simulink model "inputshaping_lab"  (R2023b)
settings: Solver=ode5  StartTime=0.0  StopTime=20  RelTol=1e-3
values from neighbouring files (symbols this model uses):
  SampleTime = 0.01    [responses0704.m]
undefined symbols (not defined in the file or in its folder): National_Instruments, PCI
libraries: sldrtlib x24, SignalEditorBlockLib x3
settings Model: Creator=labadmin  LastModifiedBy=labadmin
settings HardwareCC: ProdBitPerLong=64  ProdHWDeviceType=Intel->x86-64 (Linux 64)
settings RTWCC: Description=Simulink Desktop Real-Time  SystemTargetFile=sldrt.tlc  TemplateMakefile=sldrt.tmf  RTWCompilerOptimization=on
settings CodeAppCC: MaxIdLength=95
settings SimulinkDesktopRealTimeCC: TargetLibSuffix=_sldrt.a  TargetPreCompLibLocation=C:\Program Files\MATLAB\R2023b\toolbox\sldrt\lib\win64

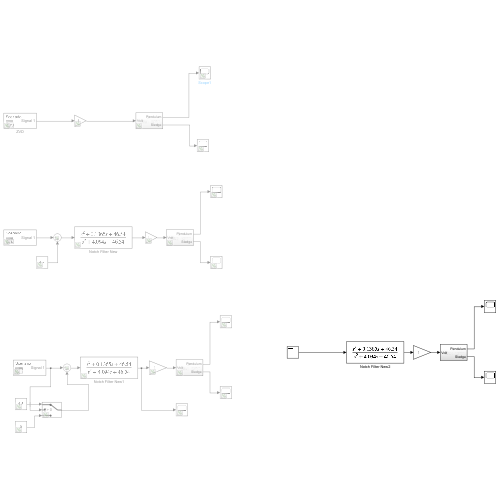
[thumbnail: Simulink's stored preview of the top-level diagram]
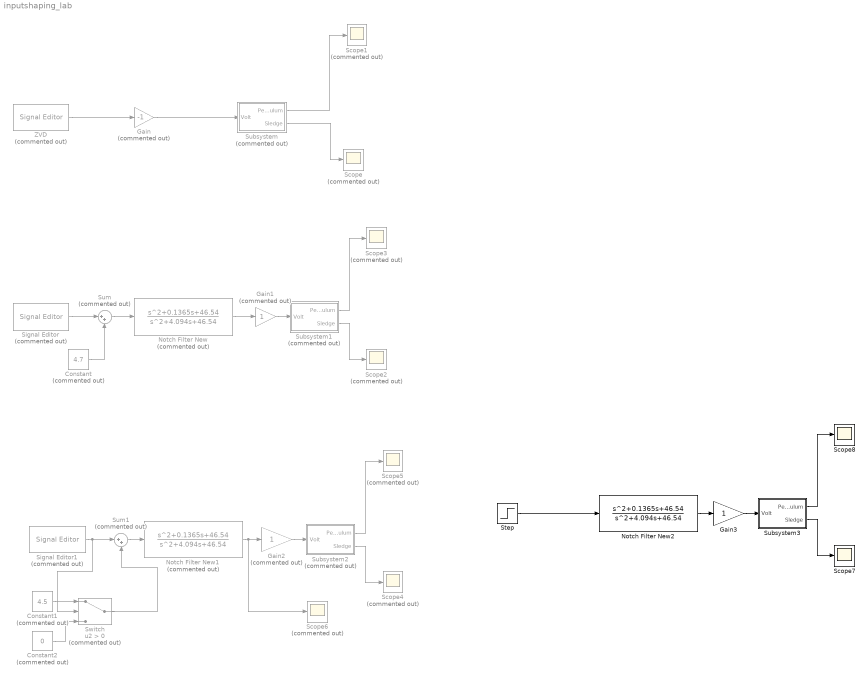
== system inputshaping_lab ==
  Constant : Constant  Commented=on  Value=4.7
  Constant1 : Constant  Commented=on  Value=4.5
  Constant2 : Constant  Commented=on  Value=0
  Gain : Gain  Commented=on  Gain=-1
  Gain1 : Gain  Commented=on
  Gain2 : Gain  Commented=on
  Gain3 : Gain
  Notch Filter New : TransferFcn  Commented=on  Numerator=[1 0.1365 46.54]  Denominator=[1 4.094 46.54]
  Notch Filter New1 : TransferFcn  Commented=on  Numerator=[1 0.1365 46.54]  Denominator=[1 4.094 46.54]
  Notch Filter New2 : TransferFcn  Numerator=[1 0.1365 46.54]  Denominator=[1 4.094 46.54]
  Scope{,1..6} (7 alike) : Scope  Commented=on
  Scope7 : Scope
  Scope8 : Scope
  Signal Editor : SignalEditorBlockLib/Signal Editor  Commented=on  FileName=ZV.mat  ActiveScenario=Scenario  ActiveSignal=Signal 1  IsBus=off  OutputBusObjectStr=Bus: BusObject  SampleTime=0  ZeroCross=off  OutputAfterFinalValue=Setting to zero  Unit=inherit  PreserveSignalName=on  ApplySigPropsToAllScenarios=on  ApplySigPropsToAllSignals=off
  Signal Editor1 : SignalEditorBlockLib/Signal Editor  Commented=on  FileName=ZV.mat  ActiveScenario=Scenario  ActiveSignal=Signal 1  IsBus=off  OutputBusObjectStr=Bus: BusObject  SampleTime=0  ZeroCross=off  OutputAfterFinalValue=Setting to zero  Unit=inherit  PreserveSignalName=on  ApplySigPropsToAllScenarios=on  ApplySigPropsToAllSignals=off
  Step : Step  Time=1.2  Before=9  After=0  SampleTime=0
  Subsystem : Subsystem  Commented=on
  Subsystem1 : Subsystem  Commented=on
  Subsystem2 : Subsystem  Commented=on
  Subsystem3 : Subsystem
  Sum : Sum  Commented=on  Inputs=|++
  Sum1 : Sum  Commented=on  Inputs=|++
  Switch : Switch  Commented=on  Criteria=u2 > Threshold  SaturateOnIntegerOverflow=off  InputSameDT=off
  ZVD : SignalEditorBlockLib/Signal Editor  Commented=on  FileName=signal_input2.mat  ActiveScenario=Scenario  ActiveSignal=Signal 1  IsBus=off  OutputBusObjectStr=Bus: BusObject  SampleTime=0  ZeroCross=off  OutputAfterFinalValue=Setting to zero  Unit=inherit  PreserveSignalName=on  ApplySigPropsToAllScenarios=on  ApplySigPropsToAllSignals=off
  wires:
  ZVD/1 -> Gain/1
  Signal Editor/1 -> Sum/1
  Subsystem/1(Pendulum) -> Scope1/1
  Subsystem/2(Sledge) -> Scope/1
  Gain/1 -> Subsystem/1(Volt)
  Notch Filter New/1 -> Gain1/1
  Subsystem1/1(Pendulum) -> Scope3/1
  Subsystem1/2(Sledge) -> Scope2/1
  Sum/1 -> Notch Filter New/1
  Constant/1 -> Sum/2
  Gain1/1 -> Subsystem1/1(Volt)
  Switch/1 -> Sum1/2
  Subsystem2/2(Sledge) -> Scope4/1
  Signal Editor1/1 -> Switch/2, Sum1/1
  Sum1/1 -> Notch Filter New1/1
  Subsystem2/1(Pendulum) -> Scope5/1
  Gain2/1 -> Subsystem2/1(Volt)
  Constant1/1 -> Switch/1
  Constant2/1 -> Switch/3
  Gain3/1 -> Subsystem3/1(Volt)
  Subsystem3/2(Sledge) -> Scope7/1
  Subsystem3/1(Pendulum) -> Scope8/1
  Step/1 -> Notch Filter New2/1
  Notch Filter New1/1 -> Scope6/1, Gain2/1
  Notch Filter New2/1 -> Gain3/1

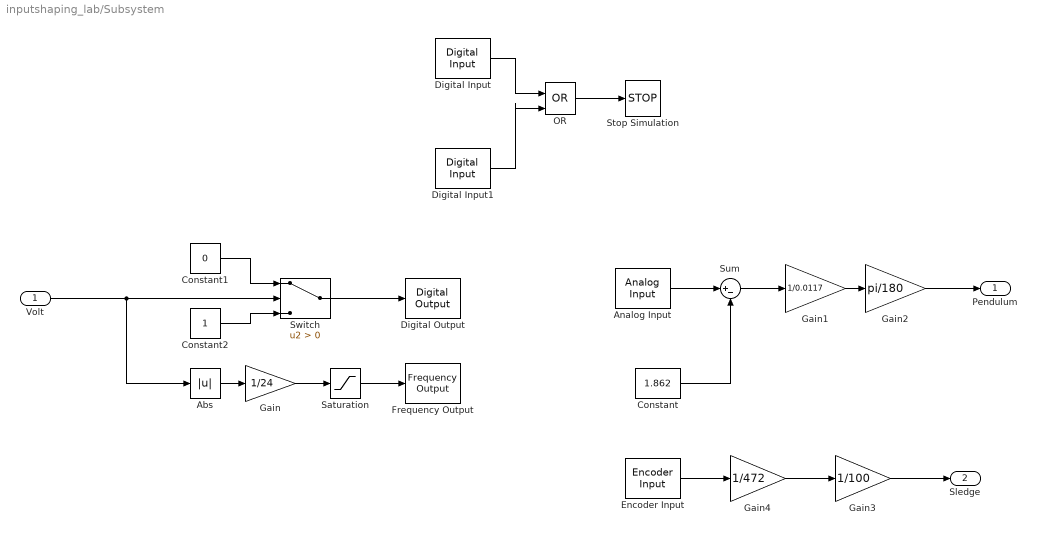
== system inputshaping_lab/Subsystem ==
  Volt : Inport
  Abs : Abs  SaturateOnIntegerOverflow=off
  Analog Input : sldrtlib/Analog Input  SampleTime=-1  MaxMissedTicks=1000000000  ShowMissedTicks=off  YieldWhenWaiting=off  DrvName=National_Instruments/PCI-6229  DrvAddress=4294967295  DrvOptions=[0 1 8192 2 3]  Channels=1  RangeMode=1  VoltRange=1  DataType=1
      settings: AttributesFormatString=National Instruments\nPCI-6229 [auto]
  Constant : Constant  Value=1.862
  Constant1 : Constant  Value=0
  Constant2 : Constant
  Digital Input : sldrtlib/Digital Input  SampleTime=0.1  MaxMissedTicks=10  ShowMissedTicks=off  YieldWhenWaiting=off  DrvName=National_Instruments/PCI-6229  DrvAddress=0  DrvOptions=[1 1 8192 2 3]  Channels=3  BitMode=1  DataType=1
      settings: AttributesFormatString=National Instruments\nPCI-6229 [0]
  Digital Input1 : sldrtlib/Digital Input  SampleTime=0.1  MaxMissedTicks=10  ShowMissedTicks=off  YieldWhenWaiting=off  DrvName=National_Instruments/PCI-6229  DrvAddress=0  DrvOptions=[1 1 8192 2 3]  Channels=2  BitMode=1  DataType=1
      settings: AttributesFormatString=National Instruments\nPCI-6229 [0]
  Digital Output : sldrtlib/Digital Output  SampleTime=-1  MaxMissedTicks=100000000  ShowMissedTicks=off  YieldWhenWaiting=off  DrvName=National_Instruments/PCI-6229  DrvAddress=4294967295  DrvOptions=[0 1 8192 2 3]  Channels=1  BitMode=1  InitialValue=[]  FinalValue=[]
      settings: AttributesFormatString=National Instruments\nPCI-6229 [auto]
  Encoder Input : sldrtlib/Encoder Input  SampleTime=-1  MaxMissedTicks=10000000  ShowMissedTicks=off  YieldWhenWaiting=off  DrvName=National_Instruments/PCI-6229  DrvAddress=4294967295  DrvOptions=[0 1 8192 2 3]  Channels=1  QuadMode=3  IndexPulse=2  InputFilter=Inf  DataType=1
      settings: AttributesFormatString=National Instruments\nPCI-6229 [auto]
  Frequency Output : sldrtlib/Frequency Output  SampleTime=-1  MaxMissedTicks=1000000000  ShowMissedTicks=off  YieldWhenWaiting=off  DrvName=National_Instruments/PCI-6229  DrvAddress=4294967295  DrvOptions=[0 1 8192 2 3]  Channels=2  FrequencySource=1  Frequency=10000  FrequencyFinalValue=[]  DutySource=2  Duty=0  DutyFinalValue=0
      settings: AttributesFormatString=National Instruments\nPCI-6229 [auto]
  Gain : Gain  Gain=1/24
  Gain1 : Gain  Gain=1/0.0117
  Gain2 : Gain  Gain=pi/180
  Gain3 : Gain  Gain=1/100
  Gain4 : Gain  Gain=1/472
  OR : Logic  Operator=OR  IconShape=distinctive  AllPortsSameDT=off  OutDataTypeStr=boolean
  Saturation : Saturate  LowerLimit=0
  Stop Simulation : Stop
  Sum : Sum  Inputs=|+-
  Switch : Switch  Criteria=u2 > Threshold  SaturateOnIntegerOverflow=off  InputSameDT=off
  Pendulum : Outport  VectorParamsAs1DForOutWhenUnconnected=off
  Sledge : Outport  Port=2  VectorParamsAs1DForOutWhenUnconnected=off
  wires:
  Abs/1 -> Gain/1
  Analog Input/1 -> Sum/1
  Gain/1 -> Saturation/1
  Volt/1 -> Abs/1, Switch/2
  Constant2/1 -> Switch/3
  Constant1/1 -> Switch/1
  Switch/1 -> Digital Output/1
  Encoder Input/1 -> Gain4/1
  Saturation/1 -> Frequency Output/1
  Sum/1 -> Gain1/1
  Gain3/1 -> Sledge/1
  Gain4/1 -> Gain3/1
  Constant/1 -> Sum/2
  Gain1/1 -> Gain2/1
  Gain2/1 -> Pendulum/1
  Digital Input1/1 -> OR/2
  Digital Input/1 -> OR/1
  OR/1 -> Stop Simulation/1

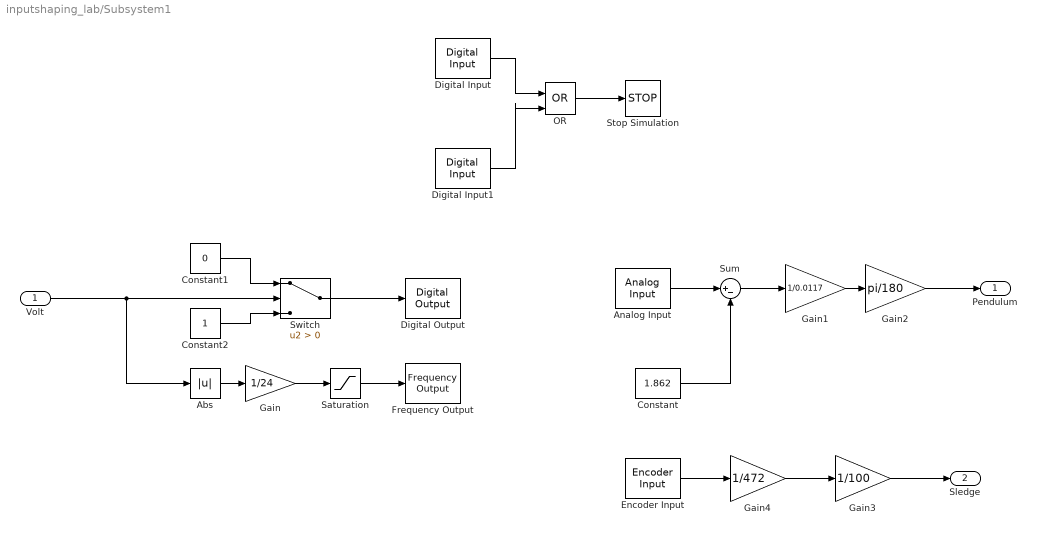
== system inputshaping_lab/Subsystem1 ==
  Volt : Inport
  Abs : Abs  SaturateOnIntegerOverflow=off
  Analog Input : sldrtlib/Analog Input  SampleTime=SampleTime  MaxMissedTicks=MaxMissedTicks  ShowMissedTicks=off  YieldWhenWaiting=off  DrvName=National_Instruments/PCI-6229  DrvAddress=4294967295  DrvOptions=[0 1 8192 2 3]  Channels=1  RangeMode=1  VoltRange=1  DataType=1
      settings: AttributesFormatString=National Instruments\nPCI-6229 [auto]
  Constant : Constant  Value=1.862
  Constant1 : Constant  Value=0
  Constant2 : Constant
  Digital Input : sldrtlib/Digital Input  SampleTime=0.1  MaxMissedTicks=10  ShowMissedTicks=off  YieldWhenWaiting=off  DrvName=National_Instruments/PCI-6229  DrvAddress=0  DrvOptions=[1 1 8192 2 3]  Channels=3  BitMode=1  DataType=1
      settings: AttributesFormatString=National Instruments\nPCI-6229 [0]
  Digital Input1 : sldrtlib/Digital Input  SampleTime=0.1  MaxMissedTicks=10  ShowMissedTicks=off  YieldWhenWaiting=off  DrvName=National_Instruments/PCI-6229  DrvAddress=0  DrvOptions=[1 1 8192 2 3]  Channels=2  BitMode=1  DataType=1
      settings: AttributesFormatString=National Instruments\nPCI-6229 [0]
  Digital Output : sldrtlib/Digital Output  SampleTime=SampleTime  MaxMissedTicks=MaxMissedTicks  ShowMissedTicks=off  YieldWhenWaiting=off  DrvName=National_Instruments/PCI-6229  DrvAddress=4294967295  DrvOptions=[0 1 8192 2 3]  Channels=1  BitMode=1  InitialValue=[]  FinalValue=[]
      settings: AttributesFormatString=National Instruments\nPCI-6229 [auto]
  Encoder Input : sldrtlib/Encoder Input  SampleTime=SampleTime  MaxMissedTicks=MaxMissedTicks  ShowMissedTicks=off  YieldWhenWaiting=off  DrvName=National_Instruments/PCI-6229  DrvAddress=4294967295  DrvOptions=[0 1 8192 2 3]  Channels=1  QuadMode=3  IndexPulse=2  InputFilter=Inf  DataType=1
      settings: AttributesFormatString=National Instruments\nPCI-6229 [auto]
  Frequency Output : sldrtlib/Frequency Output  SampleTime=SampleTime  MaxMissedTicks=MaxMissedTicks  ShowMissedTicks=off  YieldWhenWaiting=off  DrvName=National_Instruments/PCI-6229  DrvAddress=4294967295  DrvOptions=[0 1 8192 2 3]  Channels=2  FrequencySource=1  Frequency=10000  FrequencyFinalValue=[]  DutySource=2  Duty=0  DutyFinalValue=0
      settings: AttributesFormatString=National Instruments\nPCI-6229 [auto]
  Gain : Gain  Gain=1/24
  Gain1 : Gain  Gain=1/0.0117
  Gain2 : Gain  Gain=pi/180
  Gain3 : Gain  Gain=1/100
  Gain4 : Gain  Gain=1/472
  OR : Logic  Operator=OR  IconShape=distinctive  AllPortsSameDT=off  OutDataTypeStr=boolean
  Saturation : Saturate  LowerLimit=0
  Stop Simulation : Stop
  Sum : Sum  Inputs=|+-
  Switch : Switch  Criteria=u2 > Threshold  SaturateOnIntegerOverflow=off  InputSameDT=off
  Pendulum : Outport  VectorParamsAs1DForOutWhenUnconnected=off
  Sledge : Outport  Port=2  VectorParamsAs1DForOutWhenUnconnected=off
  wires:
  Abs/1 -> Gain/1
  Analog Input/1 -> Sum/1
  Gain/1 -> Saturation/1
  Volt/1 -> Abs/1, Switch/2
  Constant2/1 -> Switch/3
  Constant1/1 -> Switch/1
  Switch/1 -> Digital Output/1
  Encoder Input/1 -> Gain4/1
  Saturation/1 -> Frequency Output/1
  Sum/1 -> Gain1/1
  Gain3/1 -> Sledge/1
  Gain4/1 -> Gain3/1
  Constant/1 -> Sum/2
  Gain1/1 -> Gain2/1
  Gain2/1 -> Pendulum/1
  Digital Input1/1 -> OR/2
  Digital Input/1 -> OR/1
  OR/1 -> Stop Simulation/1

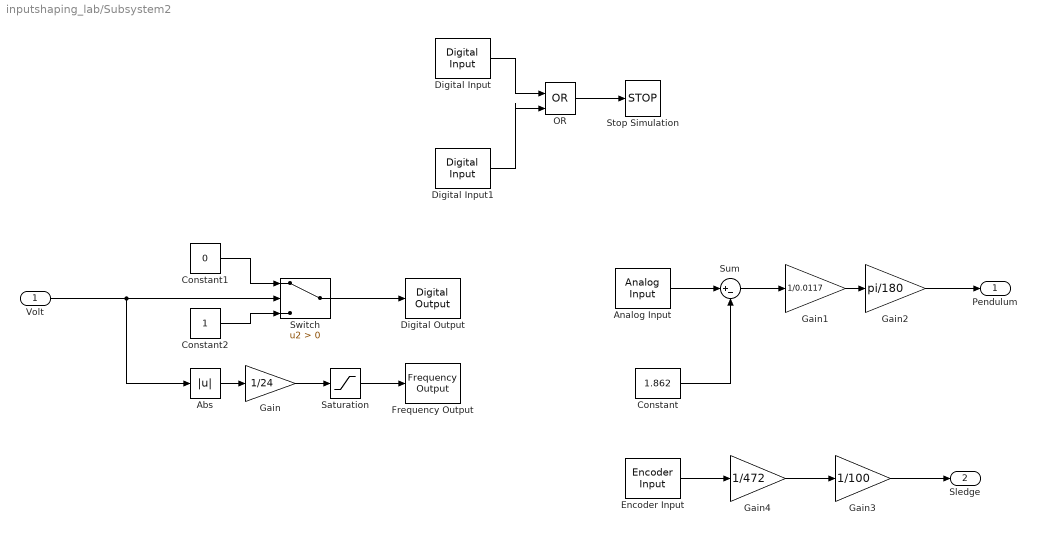
== system inputshaping_lab/Subsystem2 ==
  Volt : Inport
  Abs : Abs  SaturateOnIntegerOverflow=off
  Analog Input : sldrtlib/Analog Input  SampleTime=SampleTime  MaxMissedTicks=MaxMissedTicks  ShowMissedTicks=off  YieldWhenWaiting=off  DrvName=National_Instruments/PCI-6229  DrvAddress=4294967295  DrvOptions=[0 1 8192 2 3]  Channels=1  RangeMode=1  VoltRange=1  DataType=1
      settings: AttributesFormatString=National Instruments\nPCI-6229 [auto]
  Constant : Constant  Value=1.862
  Constant1 : Constant  Value=0
  Constant2 : Constant
  Digital Input : sldrtlib/Digital Input  SampleTime=0.1  MaxMissedTicks=10  ShowMissedTicks=off  YieldWhenWaiting=off  DrvName=National_Instruments/PCI-6229  DrvAddress=0  DrvOptions=[1 1 8192 2 3]  Channels=3  BitMode=1  DataType=1
      settings: AttributesFormatString=National Instruments\nPCI-6229 [0]
  Digital Input1 : sldrtlib/Digital Input  SampleTime=0.1  MaxMissedTicks=10  ShowMissedTicks=off  YieldWhenWaiting=off  DrvName=National_Instruments/PCI-6229  DrvAddress=0  DrvOptions=[1 1 8192 2 3]  Channels=2  BitMode=1  DataType=1
      settings: AttributesFormatString=National Instruments\nPCI-6229 [0]
  Digital Output : sldrtlib/Digital Output  SampleTime=SampleTime  MaxMissedTicks=MaxMissedTicks  ShowMissedTicks=off  YieldWhenWaiting=off  DrvName=National_Instruments/PCI-6229  DrvAddress=4294967295  DrvOptions=[0 1 8192 2 3]  Channels=1  BitMode=1  InitialValue=[]  FinalValue=[]
      settings: AttributesFormatString=National Instruments\nPCI-6229 [auto]
  Encoder Input : sldrtlib/Encoder Input  SampleTime=SampleTime  MaxMissedTicks=MaxMissedTicks  ShowMissedTicks=off  YieldWhenWaiting=off  DrvName=National_Instruments/PCI-6229  DrvAddress=4294967295  DrvOptions=[0 1 8192 2 3]  Channels=1  QuadMode=3  IndexPulse=2  InputFilter=Inf  DataType=1
      settings: AttributesFormatString=National Instruments\nPCI-6229 [auto]
  Frequency Output : sldrtlib/Frequency Output  SampleTime=SampleTime  MaxMissedTicks=MaxMissedTicks  ShowMissedTicks=off  YieldWhenWaiting=off  DrvName=National_Instruments/PCI-6229  DrvAddress=4294967295  DrvOptions=[0 1 8192 2 3]  Channels=2  FrequencySource=1  Frequency=10000  FrequencyFinalValue=[]  DutySource=2  Duty=0  DutyFinalValue=0
      settings: AttributesFormatString=National Instruments\nPCI-6229 [auto]
  Gain : Gain  Gain=1/24
  Gain1 : Gain  Gain=1/0.0117
  Gain2 : Gain  Gain=pi/180
  Gain3 : Gain  Gain=1/100
  Gain4 : Gain  Gain=1/472
  OR : Logic  Operator=OR  IconShape=distinctive  AllPortsSameDT=off  OutDataTypeStr=boolean
  Saturation : Saturate  LowerLimit=0
  Stop Simulation : Stop
  Sum : Sum  Inputs=|+-
  Switch : Switch  Criteria=u2 > Threshold  SaturateOnIntegerOverflow=off  InputSameDT=off
  Pendulum : Outport  VectorParamsAs1DForOutWhenUnconnected=off
  Sledge : Outport  Port=2  VectorParamsAs1DForOutWhenUnconnected=off
  wires:
  Abs/1 -> Gain/1
  Analog Input/1 -> Sum/1
  Gain/1 -> Saturation/1
  Volt/1 -> Abs/1, Switch/2
  Constant2/1 -> Switch/3
  Constant1/1 -> Switch/1
  Switch/1 -> Digital Output/1
  Encoder Input/1 -> Gain4/1
  Saturation/1 -> Frequency Output/1
  Sum/1 -> Gain1/1
  Gain3/1 -> Sledge/1
  Gain4/1 -> Gain3/1
  Constant/1 -> Sum/2
  Gain1/1 -> Gain2/1
  Gain2/1 -> Pendulum/1
  Digital Input1/1 -> OR/2
  Digital Input/1 -> OR/1
  OR/1 -> Stop Simulation/1

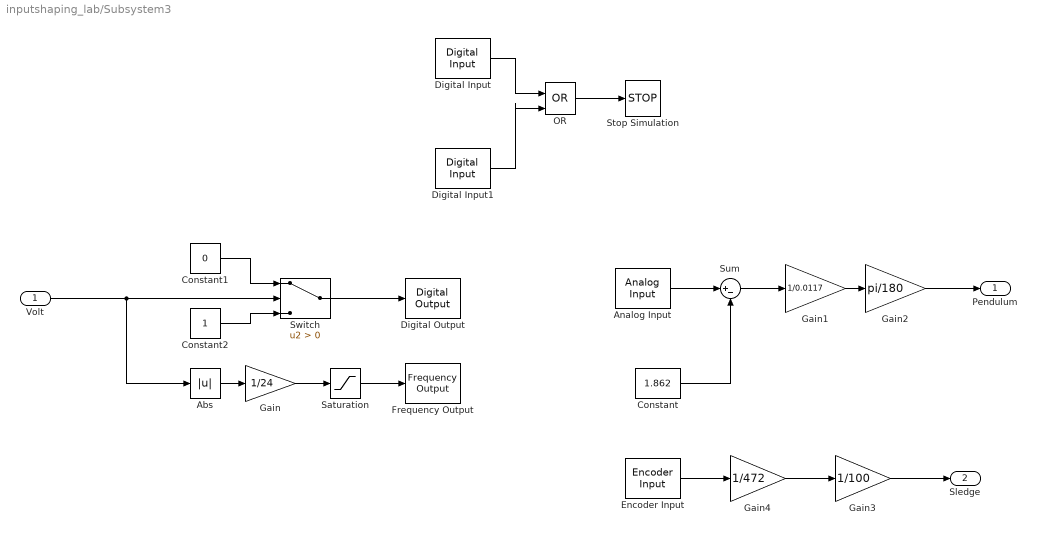
== system inputshaping_lab/Subsystem3 ==
  Volt : Inport
  Abs : Abs  SaturateOnIntegerOverflow=off
  Analog Input : sldrtlib/Analog Input  SampleTime=SampleTime  MaxMissedTicks=MaxMissedTicks  ShowMissedTicks=off  YieldWhenWaiting=off  DrvName=National_Instruments/PCI-6229  DrvAddress=4294967295  DrvOptions=[0 1 8192 2 3]  Channels=1  RangeMode=1  VoltRange=1  DataType=1
      settings: AttributesFormatString=National Instruments\nPCI-6229 [auto]
  Constant : Constant  Value=1.862
  Constant1 : Constant  Value=0
  Constant2 : Constant
  Digital Input : sldrtlib/Digital Input  SampleTime=0.1  MaxMissedTicks=10  ShowMissedTicks=off  YieldWhenWaiting=off  DrvName=National_Instruments/PCI-6229  DrvAddress=0  DrvOptions=[1 1 8192 2 3]  Channels=3  BitMode=1  DataType=1
      settings: AttributesFormatString=National Instruments\nPCI-6229 [0]
  Digital Input1 : sldrtlib/Digital Input  SampleTime=0.1  MaxMissedTicks=10  ShowMissedTicks=off  YieldWhenWaiting=off  DrvName=National_Instruments/PCI-6229  DrvAddress=0  DrvOptions=[1 1 8192 2 3]  Channels=2  BitMode=1  DataType=1
      settings: AttributesFormatString=National Instruments\nPCI-6229 [0]
  Digital Output : sldrtlib/Digital Output  SampleTime=SampleTime  MaxMissedTicks=MaxMissedTicks  ShowMissedTicks=off  YieldWhenWaiting=off  DrvName=National_Instruments/PCI-6229  DrvAddress=4294967295  DrvOptions=[0 1 8192 2 3]  Channels=1  BitMode=1  InitialValue=[]  FinalValue=[]
      settings: AttributesFormatString=National Instruments\nPCI-6229 [auto]
  Encoder Input : sldrtlib/Encoder Input  SampleTime=SampleTime  MaxMissedTicks=MaxMissedTicks  ShowMissedTicks=off  YieldWhenWaiting=off  DrvName=National_Instruments/PCI-6229  DrvAddress=4294967295  DrvOptions=[0 1 8192 2 3]  Channels=1  QuadMode=3  IndexPulse=1  InputFilter=Inf  DataType=1
      settings: AttributesFormatString=National Instruments\nPCI-6229 [auto]
  Frequency Output : sldrtlib/Frequency Output  SampleTime=SampleTime  MaxMissedTicks=MaxMissedTicks  ShowMissedTicks=off  YieldWhenWaiting=off  DrvName=National_Instruments/PCI-6229  DrvAddress=4294967295  DrvOptions=[0 1 8192 2 3]  Channels=2  FrequencySource=1  Frequency=10000  FrequencyFinalValue=[]  DutySource=2  Duty=0  DutyFinalValue=0
      settings: AttributesFormatString=National Instruments\nPCI-6229 [auto]
  Gain : Gain  Gain=1/24
  Gain1 : Gain  Gain=1/0.0117
  Gain2 : Gain  Gain=pi/180
  Gain3 : Gain  Gain=1/100
  Gain4 : Gain  Gain=1/472
  OR : Logic  Operator=OR  IconShape=distinctive  AllPortsSameDT=off  OutDataTypeStr=boolean
  Saturation : Saturate  LowerLimit=0
  Stop Simulation : Stop
  Sum : Sum  Inputs=|+-
  Switch : Switch  Criteria=u2 > Threshold  SaturateOnIntegerOverflow=off  InputSameDT=off
  Pendulum : Outport  VectorParamsAs1DForOutWhenUnconnected=off
  Sledge : Outport  Port=2  VectorParamsAs1DForOutWhenUnconnected=off
  wires:
  Abs/1 -> Gain/1
  Analog Input/1 -> Sum/1
  Gain/1 -> Saturation/1
  Volt/1 -> Abs/1, Switch/2
  Constant2/1 -> Switch/3
  Constant1/1 -> Switch/1
  Switch/1 -> Digital Output/1
  Encoder Input/1 -> Gain4/1
  Saturation/1 -> Frequency Output/1
  Sum/1 -> Gain1/1
  Gain3/1 -> Sledge/1
  Gain4/1 -> Gain3/1
  Constant/1 -> Sum/2
  Gain1/1 -> Gain2/1
  Gain2/1 -> Pendulum/1
  Digital Input1/1 -> OR/2
  Digital Input/1 -> OR/1
  OR/1 -> Stop Simulation/1
